simulink model "feb_13_p"  (R2025b)
settings: Solver=VariableStepAuto  StartTime=0.0  StopTime=6  RelTol=1e-3
libraries: spsSeriesRLCBranchLib x3, spsVoltageMeasurementLib x2, spsDCVoltageSourceLib x1, spsCurrentMeasurementLib x1, spsDiodeLib x1, spsMosfetLib x1, spspowerguiLib x1

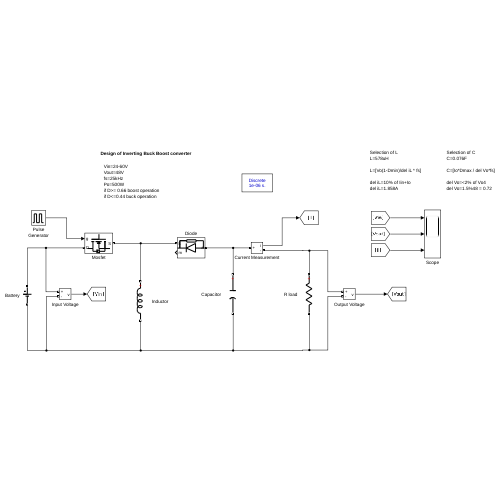
[thumbnail: Simulink's stored preview of the top-level diagram]
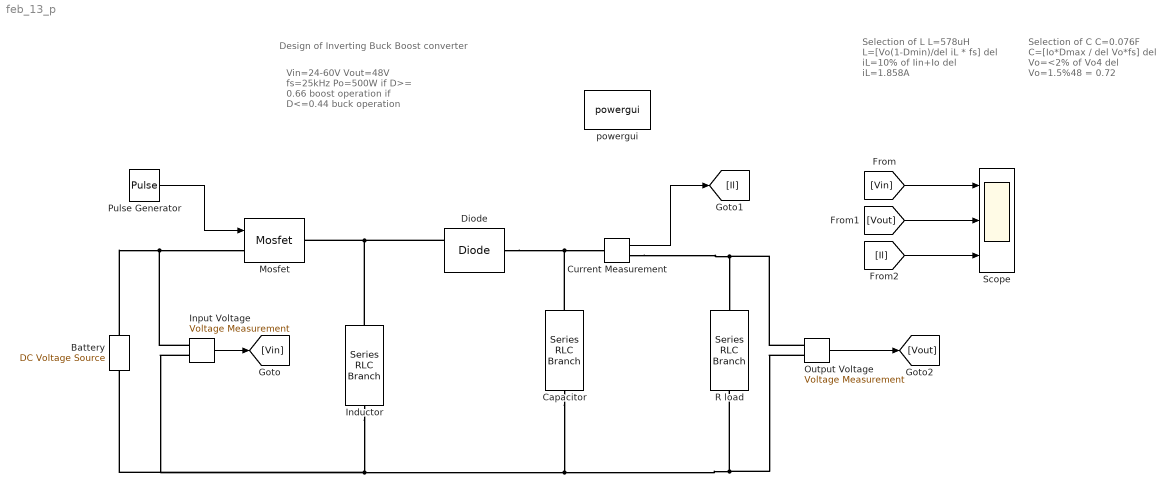
== system feb_13_p ==
  note: Vin=24-60V
      | Vout=48V
      | fs=25kHz
      | Po=500W
      | if D>= 0.66 boost operation
      | if D<=0.44 buck operation
  note: Design of Inverting Buck Boost converter
  note: Selection of C
      | C=0.076F
      |
      | C=[Io*Dmax / del Vo*fs]
      |
      | del Vo=<2% of Vo4
      | del Vo=1.5%48 = 0.72
  note: Selection of L
      | L=578uH
      |
      | L=[Vo(1-Dmin)/del iL * fs]
      |
      | del iL=10% of Iin+Io
      | del iL=1.858A
  Battery : spsDCVoltageSourceLib/DC Voltage Source  Amplitude=30  Measurements=None
  Capacitor : spsSeriesRLCBranchLib/Series RLC Branch  LConnTagsString=__new0  RConnTagsString=__new0  BranchType=C  Resistance=50  Inductance=3e-3  SetiL0=off  InitialCurrent=0  Capacitance=0.076  Setx0=off  InitialVoltage=0  Measurements=None
  Current Measurement : spsCurrentMeasurementLib/Current Measurement  PhasorSimulation=off  OutputType=Complex  PSBequivalent=0
  Diode : spsDiodeLib/Diode  Ron=0.001  Lon=0  Vf=0.8  IC=0  UseSnubber=off  Rs=50000  Cs=250e-9  Measurements=on
  Inductor : spsSeriesRLCBranchLib/Series RLC Branch  LConnTagsString=__new0  RConnTagsString=__new0  BranchType=L  Resistance=50  Inductance=578e-6  SetiL0=off  InitialCurrent=0  Capacitance=1e-6  Setx0=off  InitialVoltage=0  Measurements=None
  Input Voltage : spsVoltageMeasurementLib/Voltage Measurement  PhasorSimulation=off  OutputType=Complex  PSBequivalent=0
  Mosfet : spsMosfetLib/Mosfet  Ron=0.1  Lon=0  Rd=0.01  Vfd=0  IC=0  Rs=1e5  Cs=inf  Measurements=off
  Output Voltage : spsVoltageMeasurementLib/Voltage Measurement  PhasorSimulation=off  OutputType=Complex  PSBequivalent=0
  Pulse Generator : DiscretePulseGenerator  PulseType=Time based  Period=1/25000  PulseWidth=25
  R load : spsSeriesRLCBranchLib/Series RLC Branch  LConnTagsString=__new0  RConnTagsString=__new0  BranchType=R  Resistance=4.7  Inductance=1e-3  SetiL0=off  InitialCurrent=0  Capacitance=1e-6  Setx0=off  InitialVoltage=0  Measurements=None
  Scope : Scope  NumInputPorts=3
      settings: ActiveDisplayYMinimum=-623.44453828169662  ActiveDisplayYMaximum=281.73128002769511
  powergui : spspowerguiLib/powergui  Priority=1  SimulationMode=Discrete  SampleTime=1e-6  frequency=60  Iterations=50  frequencyindice=0  Pbase=100e6  ErrMax=1e-4  UnitsV=kV  UnitsW=MW  buscounter=0  FunctionMessages=off  echomessages=off  EnableUseOfTLC=off  CurrentSourceSwitches=off  DisableSnubberDevices=off  DisableRonSwitches=off  DisableVfSwitches=off  DisplayEquations=off  AutomaticDiscreteSolvers=off  SolverType=Tustin/Backward Euler (TBE)  Interpol=off  ExternalGateDelay=off  methode=off  Ts=10  x0status=blocks  SPID=off  SwTol=0  HookPort=off  NonlinearTolerance=1e-4  nMaxIteration=100  ContinueOnMaxIteration=off  RestoreLinks=warning  ResistiveCurrentMeasurement=off  Frange=[0:2:500]  Ylog=off  Xlog=on  ShowGrid=off  save=off  variable=ZData  structure=0  ZoomFFT=off  StartTime=0.0  cycles=1  DisplayStyle=1  fundamental=60  FreqAxis=off  MaxFrequency=1000  frequencyindicesteady=1  RmsSteady=1  display=off
  wires:
  Pulse Generator/1 -> Mosfet/1
  Current Measurement/1 -> [Il]
  Output Voltage/1 -> [Vout]
  [Vin] -> Scope/1
  Input Voltage/1 -> [Vin]
  [Vout] -> Scope/2
  [Il] -> Scope/3
  connections:
  Battery/RConn1 -- Input Voltage/LConn1 -- Mosfet/LConn1
  Capacitor/LConn1 -- Current Measurement/LConn1 -- Diode/LConn1
  Capacitor/RConn1 -- Inductor/RConn1 -- Battery/LConn1 -- Input Voltage/LConn2 -- Output Voltage/LConn2 -- R load/RConn1
  Current Measurement/RConn1 -- Output Voltage/LConn1 -- R load/LConn1
  Diode/RConn1 -- Inductor/LConn1 -- Mosfet/RConn1
